simulink model "PubIfDecisionLM_MDL"  (R2020b)
settings: configuration reference "DspaceConfig" (kept outside this file)
PostLoadFcn:
  | if any(exist('dsrtsu_mdlpostloadfcn', 'file') ~= 0), dsrtsu_mdlpostloadfcn('Execute', bdroot); end
InitFcn:
  | , if any(exist('dsmpb_private', 'file') ~= 0), dsmpb_private('dsmpb_mdlclblib', 'Init', bdroot); end,
undefined symbols (not defined in the file or in its folder): OFM_OBJ_FUSIONTYPE_E, OFM_OBJ_MOVINGSTATE_E, OFM_OBJ_ORIENTATION_E, OFM_OBJ_TYPE_E, P_LM_Cyc, P_LM_EMLHistKapRcdBufSize, P_LM_EMLHistTrajBaseDis, P_LM_EMLHistTrajPNum, P_LM_EMLKapCorrMaxThre, P_LM_EMLMinKapThre, P_LM_EMLPathDisDiffThre, P_LM_EMLQuaFiltPar, P_LM_EMLTurnActKapThre, P_LM_EMLValidQuaThre, P_LM_FntPath1Disgap, P_LM_FntPath1MinDis, P_LM_FntPath1Timegap, P_LM_FntPath2Disgap, P_LM_FntPath2MinDis, P_LM_FntPath2Timegap, P_LM_FntPath3Disgap, P_LM_FntPath3MinDis, P_LM_FntPath3Timegap, P_LM_FusBLParFiltP, P_LM_FusEVDifC2Thre, P_LM_FusEVOPath1AllVSLDisThre, P_LM_FusEVOPath1AllVSLLostNumThre, P_LM_FusEVOPath1AllVSLQuaThre, P_LM_FusEVOPath1OTLFacNLC, P_LM_FusOTLQuaThre, P_LM_FusOTLSW, P_LM_FusParC0Index, P_LM_FusParC1Index, P_LM_FusParC2Index, P_LM_FusParC3Index, P_LM_FusVSLQuaThre, P_LM_FusVSLSW, P_LM_FusVSLValidSteerWheerAngThre, P_LM_FusVSLValidVxvThre, P_LM_LaneWidth, P_LM_OTLBufTPInfoEvaFactor, P_LM_OTLObjNum, P_LM_OTLObjSelectAgeThre, P_LM_OTLObjSelectDxAssessVx, P_LM_OTLObjSelectDxThre, P_LM_OTLObjSelectVxThre, P_LM_OTLObjSelectVyAssessDx, P_LM_OTLObjSelectVyThre, P_LM_OTLTrajPntBaseDis, P_LM_OTLTrajStdThre, P_LM_VSLAvailLineNum, P_LM_VSLBLSDiffThre, P_LM_VSLBLSDisRatio, P_LM_VSLFusBLParFiltP_C1, P_LM_VSLFusBLParFiltP_C2, P_LM_VSLFusBLParFiltP_C3, P_LM_VSLFusBLParFiltP_Quality, P_LM_VSLHistTrajBaseDis, P_LM_VSLHistTrajPNum, P_LM_VSLLCC0diff ... (+18)
libraries: simulink x145, LM_LIB x43
(part 16 of 24)

== system PubIfDecisionLM_MDL/Subsystem2/LM_OTL/LM_OTL_MovObjTrajRecord3/LM_OTL_ObjStoreInfoCalc/Subsystem/LM_OTL_BufLastTPInfo/Subsystem ==
  LM_OTLBufL1LastTPValidAdju : Inport
  LM_OTLBufL1LastPNumAdju : Inport  Port=2
  LM_OTLBufL1LastSPPosAdju : Inport  Port=3
  LM_OTLBufL1LastEPPosAdju : Inport  Port=4
  LM_OTLBufL2LastTPValidAdju : Inport  Port=5
  LM_OTLBufL2LastPNumAdju : Inport  Port=6
  LM_OTLBufL2LastSPPosAdju : Inport  Port=7
  LM_OTLBufL2LastEPPosAdju : Inport  Port=8
  LM_OTLBufE1LastTPValidAdju : Inport  Port=9
  LM_OTLBufE1LastPNumAdju : Inport  Port=10
  LM_OTLBufE1LastSPPosAdju : Inport  Port=11
  LM_OTLBufE1LastEPPosAdju : Inport  Port=12
  LM_OTLBufE2LastTPValidAdju : Inport  Port=13
  LM_OTLBufE2LastPNumAdju : Inport  Port=14
  LM_OTLBufE2LastSPPosAdju : Inport  Port=15
  LM_OTLBufE2LastEPPosAdju : Inport  Port=16
  LM_OTLBufR1LastTPValidAdju : Inport  Port=17
  LM_OTLBufR1LastPNumAdju : Inport  Port=18
  LM_OTLBufR1LastSPPosAdju : Inport  Port=19
  LM_OTLBufR1LastEPPosAdju : Inport  Port=20
  LM_OTLBufR2LastTPValidAdju : Inport  Port=21
  LM_OTLBufR2LastPNumAdju : Inport  Port=22
  LM_OTLBufR2LastSPPosAdju : Inport  Port=23
  LM_OTLBufR2LastEPPosAdju : Inport  Port=24
  Bus Creator{4,7..9} (4 alike) : BusCreator  Inputs=6
  LM_OTLBufLastTPValid : Outport
  LM_OTLBufLastPNumInfo : Outport  Port=2
  LM_OTLBufLastSPPosInfo : Outport  Port=3
  LM_OTLBufLastEPPosInfo : Outport  Port=4
  wires:
  Bus Creator4/1 -> LM_OTLBufLastTPValid/1  "LM_OTLBufLastTPValid"
  LM_OTLBufR2LastTPValidAdju/1 -> Bus Creator4/6  "LM_OTLBufR2LastTPValid"
  LM_OTLBufR1LastTPValidAdju/1 -> Bus Creator4/5  "LM_OTLBufR1LastTPValid"
  LM_OTLBufE2LastTPValidAdju/1 -> Bus Creator4/4  "LM_OTLBufE2LastTPValid"
  LM_OTLBufE1LastTPValidAdju/1 -> Bus Creator4/3  "LM_OTLBufE1LastTPValid"
  LM_OTLBufL2LastTPValidAdju/1 -> Bus Creator4/2  "LM_OTLBufL2LastTPValid"
  LM_OTLBufL1LastTPValidAdju/1 -> Bus Creator4/1  "LM_OTLBufL1LastTPValid"
  LM_OTLBufL1LastPNumAdju/1 -> Bus Creator7/1  "LM_OTLBufL1LastPNum"
  LM_OTLBufL2LastPNumAdju/1 -> Bus Creator7/2  "LM_OTLBufL2LastPNum"
  LM_OTLBufE1LastPNumAdju/1 -> Bus Creator7/3  "LM_OTLBufE1LastPNum"
  LM_OTLBufE2LastPNumAdju/1 -> Bus Creator7/4  "LM_OTLBufE2LastPNum"
  LM_OTLBufR1LastPNumAdju/1 -> Bus Creator7/5  "LM_OTLBufR1LastPNum"
  LM_OTLBufR2LastPNumAdju/1 -> Bus Creator7/6  "LM_OTLBufR2LastPNum"
  LM_OTLBufL1LastSPPosAdju/1 -> Bus Creator8/1  "LM_OTLBufL1LastSPPos"
  LM_OTLBufL2LastSPPosAdju/1 -> Bus Creator8/2  "LM_OTLBufL2LastSPPos"
  LM_OTLBufE1LastSPPosAdju/1 -> Bus Creator8/3  "LM_OTLBufE1LastSPPos"
  LM_OTLBufE2LastSPPosAdju/1 -> Bus Creator8/4  "LM_OTLBufE2LastSPPos"
  LM_OTLBufR1LastSPPosAdju/1 -> Bus Creator8/5  "LM_OTLBufR1LastSPPos"
  LM_OTLBufR2LastSPPosAdju/1 -> Bus Creator8/6  "LM_OTLBufR2LastSPPos"
  LM_OTLBufR2LastEPPosAdju/1 -> Bus Creator9/6  "LM_OTLBufR2LastEPPos"
  LM_OTLBufR1LastEPPosAdju/1 -> Bus Creator9/5  "LM_OTLBufR1LastEPPos"
  LM_OTLBufE2LastEPPosAdju/1 -> Bus Creator9/4  "LM_OTLBufE2LastEPPos"
  LM_OTLBufE1LastEPPosAdju/1 -> Bus Creator9/3  "LM_OTLBufE1LastEPPos"
  LM_OTLBufL2LastEPPosAdju/1 -> Bus Creator9/2  "LM_OTLBufL2LastEPPos"
  LM_OTLBufL1LastEPPosAdju/1 -> Bus Creator9/1  "LM_OTLBufL1LastEPPos"
  Bus Creator7/1 -> LM_OTLBufLastPNumInfo/1  "LM_OTLBufLastPNumInfo"
  Bus Creator8/1 -> LM_OTLBufLastSPPosInfo/1  "LM_OTLBufLastSPPosInfo"
  Bus Creator9/1 -> LM_OTLBufLastEPPosInfo/1  "LM_OTLBufLastEPPosInfo"

== system PubIfDecisionLM_MDL/Subsystem2/LM_VSL/LM_VSLFntPath/LM_VSL_LineInfoEvalutaion/LM_VSL_BaseLinePCalc3/Subsystem/Switch Case Action Subsystem ==
  LM_VSLLineMinQualityIndex : Inport
  LM_VSLLineC1Vect : Inport  Port=2
  LM_VSLLineC2Vect : Inport  Port=3
  LM_VSLLineC3Vect : Inport  Port=4
  LM_VSLLineQualityVect : Inport  Port=5
  LM_VSLMinQualityLineValid : Inport  Port=6
  LM_VSLLineDisFntVect : Inport  Port=7
  LM_VSLBLFntDis : Inport  Port=8
  Action Port : ActionPort  ActionPortLabel=case [ 2 ]:
  LM_VSLBaseParCalc : Subsystem
  LM_VSLLineQualitySumCalc : Subsystem
  LM_VSLBaseC1 : Outport
  LM_VSLBaseC2 : Outport  Port=2
  LM_VSLBaseC3 : Outport  Port=3
  LM_VSLBaseQuality : Outport  Port=4
  wires:
  LM_VSLLineQualitySumCalc/2(Diffnum) -> LM_VSLBaseParCalc/2(Diffnum)
  LM_VSLBLFntDis/1 -> LM_VSLLineQualitySumCalc/5(LM_VSLBLFntDis)
  LM_VSLLineDisFntVect/1 -> LM_VSLLineQualitySumCalc/4(LM_VSLLineDisFntVect)
  LM_VSLMinQualityLineValid/1 -> LM_VSLLineQualitySumCalc/3(LM_VSLMinQualityLineValid), LM_VSLBaseParCalc/5(LM_VSLMinQualityLineValid)
  LM_VSLBaseParCalc/3(LM_VSLBaseC3) -> LM_VSLBaseC3/1
  LM_VSLBaseParCalc/2(LM_VSLBaseC2) -> LM_VSLBaseC2/1
  LM_VSLBaseParCalc/1(LM_VSLBaseC1) -> LM_VSLBaseC1/1
  [LM_VSLLineMinQualityIndex] -> LM_VSLBaseParCalc/3(LM_VSLLineMinQualityIndex)
  LM_VSLLineC3Vect/1 -> LM_VSLBaseParCalc/8(LM_VSLLineC3Vect)
  LM_VSLLineC2Vect/1 -> LM_VSLBaseParCalc/7(LM_VSLLineC2Vect)
  LM_VSLLineC1Vect/1 -> LM_VSLBaseParCalc/6(LM_VSLLineC1Vect)
  LM_VSLLineQualitySumCalc/1(LM_VSLLineQualitySum) -> LM_VSLBaseParCalc/1(LM_VSLLineQualitySum)
  LM_VSLLineMinQualityIndex/1 -> LM_VSLLineQualitySumCalc/1(LM_VSLLineMinQualityIndex), [LM_VSLLineMinQualityIndex]
  LM_VSLLineQualityVect/1 -> LM_VSLLineQualitySumCalc/2(LM_VSLLineQualityVect), LM_VSLBaseParCalc/4(LM_VSLLineQualityVect)
  LM_VSLBaseParCalc/4(LM_VSLBaseQuality) -> LM_VSLBaseQuality/1

== system PubIfDecisionLM_MDL/Subsystem2/LM_VSL/LM_VSLFntPath/LM_VSL_LineInfoEvalutaion/LM_VSL_BaseLinePCalc3/Subsystem/Switch Case Action Subsystem1 ==
  Action Port : ActionPort  ActionPortLabel=case [ 4 ]:
  Constant{,1..3} (4 alike) : Constant  Value=0  OutDataTypeStr=single
  LM_VSLBaseC1 : Outport
  LM_VSLBaseC2 : Outport  Port=2
  LM_VSLBaseC3 : Outport  Port=3
  LM_VSLBaseQuality : Outport  Port=4
  wires:
  Constant2/1 -> LM_VSLBaseC3/1
  Constant1/1 -> LM_VSLBaseC2/1
  Constant/1 -> LM_VSLBaseC1/1
  Constant3/1 -> LM_VSLBaseQuality/1

== system PubIfDecisionLM_MDL/Subsystem2/LM_VSL/LM_VSLFntPath/LM_VSL_LineInfoEvalutaion/LM_VSL_BaseLinePCalc3/Subsystem/Switch Case Action Subsystem2 ==
  LM_VSLLineC1Vect : Inport
  LM_VSLLineC2Vect : Inport  Port=2
  LM_VSLLineC3Vect : Inport  Port=3
  LM_VSLLineQualityVect : Inport  Port=4
  LM_VSLLineMaxQualityIndex : Inport  Port=5
  Action Port : ActionPort  ActionPortLabel=case [ 3 ]:
  1-D Lookup Table : Lookup_n-D  NumberOfTableDimensions=1  BreakpointsForDimension1=P_LM_VSLAvailLineNum  Table=P_LM_VSLLineBaseQualityRatio  InternalRulePriority=Speed  RndMeth=Simplest  InputSameDT=on
  Constant1 : Constant  OutDataTypeStr=single
  Index Vector{,1..3} (4 alike) : MultiPortSwitch  Inputs=1
  Product : Product
  Saturation : Saturate  UpperLimit=4  LowerLimit=1
  LM_VSLBaseC1 : Outport
  LM_VSLBaseC2 : Outport  Port=2
  LM_VSLBaseC3 : Outport  Port=3
  LM_VSLBaseQuality : Outport  Port=4
  wires:
  Constant1/1 -> 1-D Lookup Table/1
  Product/1 -> LM_VSLBaseQuality/1
  1-D Lookup Table/1 -> Product/2
  Saturation/1 -> Index Vector/1, Index Vector1/1, Index Vector3/1, Index Vector2/1
  Index Vector2/1 -> LM_VSLBaseC3/1  "LM_VSLBaseC3"
  Index Vector/1 -> LM_VSLBaseC1/1  "LM_VSLBaseC1"
  Index Vector1/1 -> LM_VSLBaseC2/1  "LM_VSLBaseC2"
  LM_VSLLineMaxQualityIndex/1 -> Saturation/1
  LM_VSLLineC3Vect/1 -> Index Vector2/2
  LM_VSLLineC2Vect/1 -> Index Vector1/2
  LM_VSLLineC1Vect/1 -> Index Vector/2
  LM_VSLLineQualityVect/1 -> Index Vector3/2
  Index Vector3/1 -> Product/1  "LM_VSLBaseQuality"

== system PubIfDecisionLM_MDL/Subsystem2/LM_VSL/LM_VSLFntPath/LM_VSL_LineInfoEvalutaion/LM_VSL_BaseLinePCalc3/Subsystem/Switch Case Action Subsystem3 ==
  Diffnum : Inport
  LM_VSLDiffValid : Inport  Port=2
  LM_VSLLineMinQualityIndex : Inport  Port=3
  LM_VSLLineC1Vect : Inport  Port=4
  LM_VSLLineC2Vect : Inport  Port=5
  LM_VSLLineC3Vect : Inport  Port=6
  LM_VSLLineQualityVect : Inport  Port=7
  LM_VSLMinQualityLineValid : Inport  Port=8
  Action Port : ActionPort  ActionPortLabel=case [ 0 1 ]:
  LM_VSLBaseParCalc : Subsystem
  LM_VSLLineQualitySumCalc : Subsystem
  LM_VSLBaseC1 : Outport
  LM_VSLBaseC2 : Outport  Port=2
  LM_VSLBaseC3 : Outport  Port=3
  LM_VSLBaseQuality : Outport  Port=4
  wires:
  LM_VSLLineQualityVect/1 -> LM_VSLBaseParCalc/3(LM_VSLLineQualityVect), LM_VSLLineQualitySumCalc/2(LM_VSLLineQualityVect)
  LM_VSLLineMinQualityIndex/1 -> [LM_VSLLineMinQualityIndex], LM_VSLLineQualitySumCalc/1(LM_VSLLineMinQualityIndex)
  LM_VSLLineQualitySumCalc/1(LM_VSLLineQualitySum) -> LM_VSLBaseParCalc/1(LM_VSLLineQualitySum)
  LM_VSLLineC1Vect/1 -> LM_VSLBaseParCalc/7(LM_VSLLineC1Vect)
  LM_VSLLineC2Vect/1 -> LM_VSLBaseParCalc/8(LM_VSLLineC2Vect)
  LM_VSLLineC3Vect/1 -> LM_VSLBaseParCalc/9(LM_VSLLineC3Vect)
  [LM_VSLLineMinQualityIndex] -> LM_VSLBaseParCalc/2(LM_VSLLineMinQualityIndex)
  LM_VSLBaseParCalc/1(LM_VSLBaseC1) -> LM_VSLBaseC1/1
  LM_VSLBaseParCalc/2(LM_VSLBaseC2) -> LM_VSLBaseC2/1
  LM_VSLBaseParCalc/3(LM_VSLBaseC3) -> LM_VSLBaseC3/1
  LM_VSLMinQualityLineValid/1 -> LM_VSLBaseParCalc/4(LM_VSLMinQualityLineValid), LM_VSLLineQualitySumCalc/3(LM_VSLMinQualityLineValid)
  Diffnum/1 -> LM_VSLBaseParCalc/5(Diffnum), LM_VSLLineQualitySumCalc/4(Diffnum)
  LM_VSLDiffValid/1 -> LM_VSLBaseParCalc/6(LM_VSLDiffMaxValid), LM_VSLLineQualitySumCalc/5(LM_VSLDiffValidIndex)
  LM_VSLBaseParCalc/4(LM_VSLBaseQuality) -> LM_VSLBaseQuality/1

== system PubIfDecisionLM_MDL/Subsystem2/LM_VSL/LM_VSLFntPath/LM_VSL_LineInfoEvalutaion/LM_VSL_LineInfoEvalutaion/LM_VSL_LineDisEvaluation/If Action Subsystem ==
  Action Port : ActionPort  ActionPortLabel=if(u1 == 1)
  Constant : Constant  Value=0  OutDataTypeStr=single
  Constant1 : Constant  OutDataTypeStr=uint8
  Constant2 : Constant  Value=[1;2;3;4]  OutDataTypeStr=uint8
  Constant3 : Constant  Value=0  OutDataTypeStr=single
  LM_VSLLineMaxDis : Outport
  LM_VSLLineMaxDisIndex : Outport  Port=2
  LM_VSLLineDisSortIndexVect : Outport  Port=3
  LM_VSLLineMeanDis : Outport  Port=4
  wires:
  Constant3/1 -> LM_VSLLineMeanDis/1
  Constant/1 -> LM_VSLLineMaxDis/1
  Constant1/1 -> LM_VSLLineMaxDisIndex/1
  Constant2/1 -> LM_VSLLineDisSortIndexVect/1

== system PubIfDecisionLM_MDL/Subsystem2/LM_VSL/LM_VSLFntPath/LM_VSL_LineInfoEvalutaion/LM_VSL_LineInfoEvalutaion/LM_VSL_LineDisEvaluation/If Action Subsystem1 ==
  LM_VSLLineExistVect : Inport
  LM_VSLLineDisFntVect : Inport  Port=2
  Action Port : ActionPort  ActionPortLabel=else
  Constant2 : Constant  Value=[1;2;3;4]  OutDataTypeStr=uint8
  LM_VSLLineMaxDisCalc : MATLAB Function  TreatAsAtomicUnit=on
  Terminator : Terminator
  LM_VSLLineMaxDis : Outport
  LM_VSLLineMaxDisIndex : Outport  Port=2
  LM_VSLLineDisSortIndexVect : Outport  Port=3
  LM_VSLLineMeanDis : Outport  Port=4
  wires:
  LM_VSLLineMaxDisCalc/3(LM_VSLLineMeanDis) -> LM_VSLLineMeanDis/1
  LM_VSLLineDisFntVect/1 -> LM_VSLLineMaxDisCalc/1(LM_VSLLineDisFntVect)
  LM_VSLLineExistVect/1 -> Terminator/1
  LM_VSLLineMaxDisCalc/1(LM_VSLLineMaxDis) -> LM_VSLLineMaxDis/1
  LM_VSLLineMaxDisCalc/2(LM_VSLLineMaxDisIndex) -> LM_VSLLineMaxDisIndex/1
  Constant2/1 -> LM_VSLLineDisSortIndexVect/1

== system PubIfDecisionLM_MDL/Subsystem2/LM_VSL/LM_VSLFntPath/LM_VSL_LineInfoEvalutaion/LM_VSL_LineInfoEvalutaion/LM_VSL_LineQualityEvalutaion/If Action Subsystem ==
  Action Port : ActionPort  ActionPortLabel=if(u1 == 1)
  Constant{,3,5..6} (4 alike) : Constant  Value=0  OutDataTypeStr=single
  Constant1 : Constant  OutDataTypeStr=uint8
  Constant4 : Constant  OutDataTypeStr=uint8
  LM_VSLLineMaxQuality : Outport
  LM_VSLLineMaxQualityIndex : Outport  Port=2
  LM_VSLLineMinQualityIndex : Outport  Port=3
  LM_VSLLineMinQuality : Outport  Port=4
  LM_VSLLineMeanQuality : Outport  Port=5
  LM_VSLLineQualityVar : Outport  Port=6
  wires:
  Constant/1 -> LM_VSLLineMaxQuality/1
  Constant1/1 -> LM_VSLLineMaxQualityIndex/1
  Constant3/1 -> LM_VSLLineMinQuality/1
  Constant4/1 -> LM_VSLLineMinQualityIndex/1
  Constant5/1 -> LM_VSLLineMeanQuality/1
  Constant6/1 -> LM_VSLLineQualityVar/1

== system PubIfDecisionLM_MDL/Subsystem2/LM_VSL/LM_VSLFntPath/LM_VSL_LineInfoEvalutaion/LM_VSL_LineInfoEvalutaion/LM_VSL_LineQualityEvalutaion/If Action Subsystem1 ==
  LM_VSLLineExistVect : Inport
  LM_VSLLineQualityVect : Inport  Port=2
  Action Port : ActionPort  ActionPortLabel=else
  Data Type Conversion : DataTypeConversion
  For Iterator Subsystem : Subsystem  TreatAsAtomicUnit=on
  LM_VSL_LineQualityEvaluation : MATLAB Function  TreatAsAtomicUnit=on
  Terminator : Terminator
  Terminator1 : Terminator
  LM_VSLLineMaxQuality : Outport
  LM_VSLLineMaxQualityIndex : Outport  Port=2
  LM_VSLLineMinQualityIndex : Outport  Port=3
  LM_VSLLineMinQuality : Outport  Port=4
  LM_VSLLineMeanQuality : Outport  Port=5
  LM_VSLLineQualityVar : Outport  Port=6
  wires:
  LM_VSL_LineQualityEvaluation/4(LM_VSLLineMinQualiyIndex) -> Terminator1/1
  LM_VSL_LineQualityEvaluation/3(LM_VSLLineMinQualiy) -> Terminator/1
  Data Type Conversion/1 -> LM_VSLLineMinQualityIndex/1
  LM_VSLLineExistVect/1 -> LM_VSL_LineQualityEvaluation/1(LM_VSLLineExistVect)
  LM_VSL_LineQualityEvaluation/1(LM_VSLLineMaxQualiy) -> LM_VSLLineMaxQuality/1
  LM_VSL_LineQualityEvaluation/2(LM_VSLLineMaxQualiyIndex) -> LM_VSLLineMaxQualityIndex/1
  LM_VSL_LineQualityEvaluation/5(LM_VSLLineMeanQuality) -> LM_VSLLineMeanQuality/1
  LM_VSL_LineQualityEvaluation/6(LM_VSLLineQualityVar) -> LM_VSLLineQualityVar/1
  LM_VSLLineQualityVect/1 -> For Iterator Subsystem/1(LM_VSLLineQualityVect), LM_VSL_LineQualityEvaluation/2(LM_VSLLineQualityVect)
  For Iterator Subsystem/2(LM_VSLLineMinQualityIndex) -> Data Type Conversion/1
  For Iterator Subsystem/1(LM_VSLLineMinQuality) -> LM_VSLLineMinQuality/1

== system PubIfDecisionLM_MDL/Subsystem2/LM_VSL/LM_VSLFntPath/LM_VSL_LineInfoEvalutaion/LM_VSL_LineInfoEvalutaion/LM_VSL_LineQualityEvalutaion/LM_VSLMinQualityLineValidJudge ==
  LM_VSLLineMinQuality : Inport
  LM_VSLLineMeanQuality : Inport  Port=2
  Constant : Constant  Value=P_LM_VSLLineQualitydiffThre  OutDataTypeStr=single
  Constant1 : Constant  Value=P_LM_VSLLineMinQualityThre  OutDataTypeStr=single
  Logical Operator : Logic  AllPortsSameDT=off  OutDataTypeStr=boolean
  Relational Operator : RelationalOperator  Operator=<=  OutDataTypeStr=boolean  RndMeth=Nearest
  Relational Operator1 : RelationalOperator  Operator=>  OutDataTypeStr=boolean  RndMeth=Nearest
  Subtract : Sum  Inputs=+-
  LM_VSLMinQualityLineValid : Outport
  wires:
  LM_VSLLineMeanQuality/1 -> Subtract/1
  LM_VSLLineMinQuality/1 -> Relational Operator1/1, Subtract/2
  Subtract/1 -> Relational Operator/1
  Constant/1 -> Relational Operator/2
  Relational Operator/1 -> Logical Operator/1
  Constant1/1 -> Relational Operator1/2
  Relational Operator1/1 -> Logical Operator/2
  Logical Operator/1 -> LM_VSLMinQualityLineValid/1  "LM_VSLMinQualityLineValid"

== system PubIfDecisionLM_MDL/Subsystem2/LM_VSL/LM_VSLRearPath/LM_VSLHistLineInfoCoordinateConvert/If Action Subsystem/For Each Subsystem/LM_VSL_LRC0HistInfoConvert ==
  LM_VSLLRC0HistInfoXK1 : Inport
  LM_VSLLRC0HistInfoYK1 : Inport  Port=2
  LM_EgoVehOffsetX : Inport  Port=3
  LM_EgoVehOffsetY : Inport  Port=4
  LM_EgoVehOffsetAng : Inport  Port=5
  Add : Sum
  Product{,1..3} (4 alike) : Product
  Sin : Trigonometry
  Sin1 : Trigonometry  Operator=cos
  Subtract : Sum  Inputs=+-
  Subtract1 : Sum  Inputs=+-
  Subtract2 : Sum  Inputs=+-
  LM_VSLLLC0HistInfoXK1Adju : Outport
  LM_VSLLLC0HistInfoYK1Adju : Outport  Port=2
  wires:
  Subtract2/1 -> LM_VSLLLC0HistInfoXK1Adju/1  "LM_VSLLLC0HistInfoXK1Adju"
  LM_EgoVehOffsetX/1 -> Subtract/2
  LM_EgoVehOffsetY/1 -> Subtract1/2
  LM_VSLLRC0HistInfoXK1/1 -> Subtract/1
  Add/1 -> LM_VSLLLC0HistInfoYK1Adju/1  "LM_VSLLLC0HistInfoYK1Adju"
  Product3/1 -> Add/2
  Subtract/1 -> Product/1, Product2/1
  Sin/1 -> Product1/2, Product2/2
  LM_EgoVehOffsetAng/1 -> Sin/1, Sin1/1
  LM_VSLLRC0HistInfoYK1/1 -> Subtract1/1
  Product1/1 -> Subtract2/2
  Product/1 -> Subtract2/1
  Product2/1 -> Add/1
  Sin1/1 -> Product/2, Product3/2
  Subtract1/1 -> Product1/1, Product3/1

== system PubIfDecisionLM_MDL/Subsystem2/LM_VSL/LM_VSLRearPath/LM_VSLHistLineInfoCoordinateConvert/If Action Subsystem/For Each Subsystem/LM_VSL_RLC0HistInfoConvert ==
  LM_VSLRLC0HistInfoXK1 : Inport
  LM_VSLRLC0HistInfoYK1 : Inport  Port=2
  LM_EgoVehOffsetX : Inport  Port=3
  LM_EgoVehOffsetY : Inport  Port=4
  LM_EgoVehOffsetAng : Inport  Port=5
  Add : Sum
  Product{,1..3} (4 alike) : Product
  Sin : Trigonometry
  Sin1 : Trigonometry  Operator=cos
  Subtract : Sum  Inputs=+-
  Subtract1 : Sum  Inputs=+-
  Subtract2 : Sum  Inputs=+-
  LM_VSLLLC0HistInfoXK1Adju : Outport
  LM_VSLLLC0HistInfoYK1Adju : Outport  Port=2
  wires:
  Subtract1/1 -> Product3/1, Product1/1
  Sin1/1 -> Product3/2, Product/2
  Product2/1 -> Add/1
  Product/1 -> Subtract2/1
  Product1/1 -> Subtract2/2
  LM_VSLRLC0HistInfoYK1/1 -> Subtract1/1
  LM_EgoVehOffsetAng/1 -> Sin1/1, Sin/1
  Sin/1 -> Product2/2, Product1/2
  Subtract/1 -> Product2/1, Product/1
  Product3/1 -> Add/2
  Add/1 -> LM_VSLLLC0HistInfoYK1Adju/1  "LM_VSLLLC0HistInfoYK1Adju"
  LM_VSLRLC0HistInfoXK1/1 -> Subtract/1
  LM_EgoVehOffsetY/1 -> Subtract1/2
  LM_EgoVehOffsetX/1 -> Subtract/2
  Subtract2/1 -> LM_VSLLLC0HistInfoXK1Adju/1  "LM_VSLLLC0HistInfoXK1Adju"

== system PubIfDecisionLM_MDL/Subsystem2/DIR/DrivingIntentionRecognition1/DIR_LaneChangeProbCalc/DIR_LaneChangeLeftProbCalc/If Action Subsystem/DIR_LaneChgLeProbByLaneInfo/DIR_LaneC0DifCalc ==
  DIR_LaneC0DifK1 : Inport
  LM_LRC0 : Inport  Port=2
  LM_RLC0 : Inport  Port=3
  Abs : Abs
  Add : Sum
  Add1 : Sum
  Constant : Constant  Value=0.5  OutDataTypeStr=single
  Product : Product
  Subtract : Sum  Inputs=+-
  DIR_LaneC0Dif : Outport
  wires:
  Abs/1 -> Subtract/1
  Product/1 -> Add1/1
  Add/1 -> Abs/1
  LM_LRC0/1 -> Add/1
  LM_RLC0/1 -> Add/2
  DIR_LaneC0DifK1/1 -> Add1/2, Subtract/2
  Subtract/1 -> Product/1
  Constant/1 -> Product/2
  Add1/1 -> DIR_LaneC0Dif/1

== system PubIfDecisionLM_MDL/Subsystem2/DIR/DrivingIntentionRecognition1/DIR_LaneChangeProbCalc/DIR_LaneChangeLeftProbCalc/If Action Subsystem/DIR_LaneChgLeProbByLaneInfo/DIR_LaneChgLeProbCalcByLaneBorder ==
  DIR_LaneC0Dif : Inport
  LM_LRC0 : Inport  Port=2
  1-D Lookup Table : Lookup_n-D  NumberOfTableDimensions=1  BreakpointsForDimension1=single([0.7,0.79,0.88,0.97,1.06,1.15]);  Table=single([0,0.2,0.4,0.6,0.8,1]);  InternalRulePriority=Speed  RndMeth=Simplest  InputSameDT=on
  Constant : Constant  Value=1.15  OutDataTypeStr=single
  Constant1 : Constant  OutDataTypeStr=single
  Constant2 : Constant  Value=0.7  OutDataTypeStr=single
  Constant3 : Constant  Value=0  OutDataTypeStr=single
  Constant4 : Constant  Value=1.7  OutDataTypeStr=single
  Logical Operator : Logic  Inputs=3  AllPortsSameDT=off  OutDataTypeStr=boolean
  Logical Operator1 : Logic  AllPortsSameDT=off  OutDataTypeStr=boolean
  Relational Operator : RelationalOperator  OutDataTypeStr=boolean  RndMeth=Simplest
  Relational Operator1 : RelationalOperator  Operator=<  OutDataTypeStr=boolean  RndMeth=Simplest
  Relational Operator2 : RelationalOperator  OutDataTypeStr=boolean  RndMeth=Simplest
  Relational Operator3 : RelationalOperator  Operator=<  OutDataTypeStr=boolean  RndMeth=Simplest
  Switch : Switch  Criteria=u2 ~= 0
  Switch1 : Switch  Criteria=u2 ~= 0
  DIR_LC2LeProbByLaneBorder : Outport
  wires:
  Constant/1 -> Relational Operator/2, Relational Operator1/2
  Relational Operator/1 -> Logical Operator1/2
  Constant1/1 -> Switch/1
  Relational Operator1/1 -> Logical Operator/2
  Constant2/1 -> Relational Operator2/2
  Relational Operator2/1 -> Logical Operator/3
  Logical Operator/1 -> Switch1/2
  Switch1/1 -> Switch/3
  Constant3/1 -> Switch1/3
  Switch/1 -> DIR_LC2LeProbByLaneBorder/1  "DIR_LC2LeProbByLaneBorder"
  DIR_LaneC0Dif/1 -> 1-D Lookup Table/1, Relational Operator2/1, Relational Operator1/1, Relational Operator/1
  1-D Lookup Table/1 -> Switch1/1
  LM_LRC0/1 -> Relational Operator3/1
  Constant4/1 -> Relational Operator3/2
  Relational Operator3/1 -> Logical Operator/1, Logical Operator1/1
  Logical Operator1/1 -> Switch/2

== system PubIfDecisionLM_MDL/Subsystem2/DIR/DrivingIntentionRecognition1/DIR_LaneChangeProbCalc/DIR_LaneChangeLeftProbCalc/If Action Subsystem/DIR_LaneChgLeProbCalcBySteer/DIR_LaneChg2LeftProbCalcBySteer ==
  DIR_LC2LeProbBySteerWheelAng : Inport
  DIR_LC2LeProbBytTurnLamp : Inport  Port=2
  Max : MinMax  Function=max  Inputs=2
  DIR_LC2LeProbBySteer : Outport
  wires:
  DIR_LC2LeProbBySteerWheelAng/1 -> Max/1
  DIR_LC2LeProbBytTurnLamp/1 -> Max/2
  Max/1 -> DIR_LC2LeProbBySteer/1  "DIR_LC2LeProbBySteer"

== system PubIfDecisionLM_MDL/Subsystem2/DIR/DrivingIntentionRecognition1/DIR_LaneChangeProbCalc/DIR_LaneChangeLeftProbCalc/If Action Subsystem/DIR_LaneChgLeProbCalcBySteer/DIR_LaneChg2LeftProbCalcBySteerWheelAng ==
  SteerWheelAngle : Inport
  SteerWheelAngleSign : Inport  Port=2
  1-D Lookup Table : Lookup_n-D  NumberOfTableDimensions=1  BreakpointsForDimension1=single([9,15,20,25]);  Table=single([0,0.33000001311302185,0.6700000166893005,1]);  InternalRulePriority=Speed  RndMeth=Simplest  InputSameDT=on
  Constant : Constant  Value=25  OutDataTypeStr=single
  Constant1 : Constant  OutDataTypeStr=single
  Constant2 : Constant  Value=9  OutDataTypeStr=single
  Constant3 : Constant  Value=0  OutDataTypeStr=single
  Constant4 : Constant  Value=0  OutDataTypeStr=uint8
  Display{,1..3} (4 alike) : Display
  Logical Operator : Logic  Inputs=3  AllPortsSameDT=off  OutDataTypeStr=boolean
  Logical Operator1 : Logic  AllPortsSameDT=off  OutDataTypeStr=boolean
  Relational Operator : RelationalOperator  OutDataTypeStr=boolean  RndMeth=Simplest
  Relational Operator1 : RelationalOperator  Operator=<  OutDataTypeStr=boolean  RndMeth=Simplest
  Relational Operator2 : RelationalOperator  OutDataTypeStr=boolean  RndMeth=Simplest
  Relational Operator3 : RelationalOperator  Operator===  OutDataTypeStr=boolean  RndMeth=Simplest
  Switch : Switch  Criteria=u2 ~= 0
  Switch1 : Switch  Criteria=u2 ~= 0
  DIR_LC2LeProbBySteerWheelAng : Outport
  wires:
  1-D Lookup Table/1 -> Display/1, Switch1/1
  Constant/1 -> Relational Operator/2, Relational Operator1/2
  SteerWheelAngle/1 -> 1-D Lookup Table/1, Relational Operator2/1, Relational Operator1/1, Relational Operator/1
  Switch1/1 -> Display1/1, Switch/3
  Constant2/1 -> Relational Operator2/2
  Logical Operator/1 -> Display2/1, Switch1/2
  Constant3/1 -> Switch1/3
  Relational Operator1/1 -> Logical Operator/1
  Relational Operator2/1 -> Logical Operator/2
  Switch/1 -> DIR_LC2LeProbBySteerWheelAng/1  "DIR_LC2LeProbBySteerWheelAng"
  Constant1/1 -> Switch/1
  Logical Operator1/1 -> Switch/2
  SteerWheelAngleSign/1 -> Relational Operator3/1
  Relational Operator3/1 -> Display3/1, [SteerLeftFlg], Logical Operator1/1
  [SteerLeftFlg] -> Logical Operator/3
  Relational Operator/1 -> Logical Operator1/2
  Constant4/1 -> Relational Operator3/2

== system PubIfDecisionLM_MDL/Subsystem2/DIR/DrivingIntentionRecognition1/DIR_LaneChangeProbCalc/DIR_LaneChangeLeftProbCalc/If Action Subsystem/DIR_LaneChgLeProbCalcBySteer/DIR_LaneChg2LeftProbCalcByTurnLampOnTime ==
  DIR_LeftTurnLampOnTime : Inport
  1-D Lookup Table : Lookup_n-D  NumberOfTableDimensions=1  BreakpointsForDimension1=single([0,0.30000001192092896,0.6000000238418579,0.8999999761581421,1.2000000476837158,1.5]);  Table=single([0,0.20000000298023224,0.4000000059604645,0.6000000238418579,0.800000011920929,1]);  InternalRulePriority=Speed  RndMeth=Simplest  InputSameDT=on
  Constant : Constant  Value=1.5  OutDataTypeStr=single
  Constant1 : Constant  OutDataTypeStr=single
  Constant2 : Constant  Value=0  OutDataTypeStr=single
  Constant3 : Constant  Value=0  OutDataTypeStr=single
  Logical Operator : Logic  AllPortsSameDT=off  OutDataTypeStr=boolean
  Relational Operator : RelationalOperator  OutDataTypeStr=boolean  RndMeth=Simplest
  Relational Operator1 : RelationalOperator  Operator=<  OutDataTypeStr=boolean  RndMeth=Simplest
  Relational Operator2 : RelationalOperator  Operator=>  OutDataTypeStr=boolean  RndMeth=Simplest
  Switch : Switch  Criteria=u2 ~= 0
  Switch1 : Switch  Criteria=u2 ~= 0
  DIR_LC2LeProbBytTurnLamp : Outport
  wires:
  DIR_LeftTurnLampOnTime/1 -> 1-D Lookup Table/1, Relational Operator2/1, Relational Operator1/1, Relational Operator/1
  Constant/1 -> Relational Operator1/2, Relational Operator/2
  Relational Operator/1 -> Switch/2
  Constant1/1 -> Switch/1
  Constant2/1 -> Relational Operator2/2
  Relational Operator1/1 -> Logical Operator/1
  Relational Operator2/1 -> Logical Operator/2
  Logical Operator/1 -> Switch1/2
  Constant3/1 -> Switch1/3
  Switch1/1 -> Switch/3
  Switch/1 -> DIR_LC2LeProbBytTurnLamp/1  "DIR_LC2LeProbBytTurnLamp"
  1-D Lookup Table/1 -> Switch1/1

== system PubIfDecisionLM_MDL/Subsystem2/DIR/DrivingIntentionRecognition1/DIR_LaneChangeProbCalc/DIR_LaneChangeLeftProbCalc/If Action Subsystem1/DIR_LaneChgLeProbCalcBySteer/If Action Subsystem ==
  SteerWheelAngle : Inport
  SteerWheelAngleSign : Inport  Port=2
  vxvRefMs : Inport  Port=3
  Action Port : ActionPort  ActionPortLabel=if(u1 ~= 0)
  Constant1 : Constant  Value=0  OutDataTypeStr=single
  Constant2 : Constant  Value=3.5  OutDataTypeStr=single
  Constant4 : Constant  Value=0  OutDataTypeStr=uint8
  Logical Operator1 : Logic  Inputs=3  AllPortsSameDT=off  OutDataTypeStr=boolean
  Relational Operator : RelationalOperator  OutDataTypeStr=boolean  RndMeth=Simplest
  Relational Operator1 : RelationalOperator  Operator=>  OutDataTypeStr=boolean  RndMeth=Simplest
  Relational Operator3 : RelationalOperator  Operator===  OutDataTypeStr=boolean  RndMeth=Simplest
  DIR_LaneChgLeBySteerValid : Outport
  wires:
  Constant4/1 -> Relational Operator3/2
  Relational Operator3/1 -> Logical Operator1/1
  SteerWheelAngle/1 -> Relational Operator/1
  SteerWheelAngleSign/1 -> Relational Operator3/1
  Relational Operator/1 -> Logical Operator1/2
  vxvRefMs/1 -> Relational Operator1/1
  Constant2/1 -> Relational Operator/2
  Logical Operator1/1 -> DIR_LaneChgLeBySteerValid/1  "DIR_LaneChgLeBySteerValid"
  Constant1/1 -> Relational Operator1/2
  Relational Operator1/1 -> Logical Operator1/3

== system PubIfDecisionLM_MDL/Subsystem2/DIR/DrivingIntentionRecognition1/DIR_LaneChangeProbCalc/DIR_LaneChangeLeftProbCalc/If Action Subsystem1/DIR_LaneChgLeProbCalcBySteer/If Action Subsystem1 ==
  SteerWheelAngle : Inport
  SteerWheelAngleSign : Inport  Port=2
  vxvRefMs : Inport  Port=3
  Action Port : ActionPort  ActionPortLabel=else
  1-D Lookup Table : Lookup_n-D  NumberOfTableDimensions=1  BreakpointsForDimension1=single([5,15,25,35]);  Table=single([10,9,6,3]);  InternalRulePriority=Speed  RndMeth=Simplest  InputSameDT=on
  Constant1 : Constant  Value=0  OutDataTypeStr=single
  Constant4 : Constant  Value=0  OutDataTypeStr=uint8
  Logical Operator1 : Logic  Inputs=3  AllPortsSameDT=off  OutDataTypeStr=boolean
  Relational Operator : RelationalOperator  OutDataTypeStr=boolean  RndMeth=Simplest
  Relational Operator2 : RelationalOperator  Operator=>  OutDataTypeStr=boolean  RndMeth=Simplest
  Relational Operator3 : RelationalOperator  Operator===  OutDataTypeStr=boolean  RndMeth=Simplest
  DIR_LaneChgLeBySteerValid : Outport
  wires:
  Logical Operator1/1 -> DIR_LaneChgLeBySteerValid/1  "DIR_LaneChgLeBySteerValid"
  Constant4/1 -> Relational Operator3/2
  1-D Lookup Table/1 -> Relational Operator/2
  SteerWheelAngleSign/1 -> Relational Operator3/1
  SteerWheelAngle/1 -> Relational Operator/1
  Relational Operator/1 -> Logical Operator1/2
  Relational Operator3/1 -> Logical Operator1/1
  vxvRefMs/1 -> Relational Operator2/1, 1-D Lookup Table/1
  Constant1/1 -> Relational Operator2/2
  Relational Operator2/1 -> Logical Operator1/3

== system PubIfDecisionLM_MDL/Subsystem2/DIR/DrivingIntentionRecognition1/DIR_LaneChangeProbCalc/DIR_LaneChangeRightProbCalc/If Action Subsystem/DIR_LaneChgLeProbByLaneInfo/DIR_LaneC0DifCalc ==
  DIR_LaneC0DifK1 : Inport
  LM_LRC0 : Inport  Port=2
  LM_RLC0 : Inport  Port=3
  Abs : Abs
  Add : Sum
  Add1 : Sum
  Constant : Constant  Value=0.5  OutDataTypeStr=single
  Product : Product
  Subtract : Sum  Inputs=+-
  DIR_LaneC0Dif : Outport
  wires:
  Add1/1 -> DIR_LaneC0Dif/1
  Constant/1 -> Product/2
  Subtract/1 -> Product/1
  DIR_LaneC0DifK1/1 -> Subtract/2, Add1/2
  LM_RLC0/1 -> Add/2
  LM_LRC0/1 -> Add/1
  Add/1 -> Abs/1
  Product/1 -> Add1/1
  Abs/1 -> Subtract/1

== system PubIfDecisionLM_MDL/Subsystem2/DIR/DrivingIntentionRecognition1/DIR_LaneChangeProbCalc/DIR_LaneChangeRightProbCalc/If Action Subsystem/DIR_LaneChgLeProbByLaneInfo/DIR_LaneChgLeProbCalcByLaneBorder ==
  DIR_LaneC0Dif : Inport
  LM_LRC0 : Inport  Port=2
  1-D Lookup Table : Lookup_n-D  NumberOfTableDimensions=1  BreakpointsForDimension1=single([0.7,0.79,0.88,0.97,1.06,1.15]);  Table=single([0,0.2,0.4,0.6,0.8,1]);  InternalRulePriority=Speed  RndMeth=Simplest  InputSameDT=on
  Constant : Constant  Value=1.15  OutDataTypeStr=single
  Constant1 : Constant  OutDataTypeStr=single
  Constant2 : Constant  Value=0.7  OutDataTypeStr=single
  Constant3 : Constant  Value=0  OutDataTypeStr=single
  Constant4 : Constant  Value=1.7  OutDataTypeStr=single
  Logical Operator : Logic  Inputs=3  AllPortsSameDT=off  OutDataTypeStr=boolean
  Logical Operator1 : Logic  AllPortsSameDT=off  OutDataTypeStr=boolean
  Relational Operator : RelationalOperator  OutDataTypeStr=boolean  RndMeth=Simplest
  Relational Operator1 : RelationalOperator  Operator=<  OutDataTypeStr=boolean  RndMeth=Simplest
  Relational Operator2 : RelationalOperator  OutDataTypeStr=boolean  RndMeth=Simplest
  Relational Operator3 : RelationalOperator  Operator=<  OutDataTypeStr=boolean  RndMeth=Simplest
  Switch : Switch  Criteria=u2 ~= 0
  Switch1 : Switch  Criteria=u2 ~= 0
  DIR_LC2RigProbByLaneBorder : Outport
  wires:
  Logical Operator1/1 -> Switch/2
  Relational Operator3/1 -> Logical Operator1/1, Logical Operator/1
  Constant4/1 -> Relational Operator3/2
  LM_LRC0/1 -> Relational Operator3/1
  1-D Lookup Table/1 -> Switch1/1
  DIR_LaneC0Dif/1 -> Relational Operator/1, Relational Operator1/1, Relational Operator2/1, 1-D Lookup Table/1
  Switch/1 -> DIR_LC2RigProbByLaneBorder/1  "DIR_LC2RigProbByLaneBorder"
  Constant3/1 -> Switch1/3
  Switch1/1 -> Switch/3
  Logical Operator/1 -> Switch1/2
  Relational Operator2/1 -> Logical Operator/3
  Constant2/1 -> Relational Operator2/2
  Relational Operator1/1 -> Logical Operator/2
  Constant1/1 -> Switch/1
  Relational Operator/1 -> Logical Operator1/2
  Constant/1 -> Relational Operator1/2, Relational Operator/2

== system PubIfDecisionLM_MDL/Subsystem2/DIR/DrivingIntentionRecognition1/DIR_LaneChangeProbCalc/DIR_LaneChangeRightProbCalc/If Action Subsystem/DIR_LaneChgLeProbCalcBySteer/DIR_LaneChg2LeftProbCalcBySteer ==
  DIR_LC2RigProbBySteerWheelAng : Inport
  DIR_LC2RigProbBytTurnLamp : Inport  Port=2
  Max : MinMax  Function=max  Inputs=2
  DIR_LC2RigProbBySteer : Outport
  wires:
  Max/1 -> DIR_LC2RigProbBySteer/1  "DIR_LC2RigProbBySteer"
  DIR_LC2RigProbBytTurnLamp/1 -> Max/2
  DIR_LC2RigProbBySteerWheelAng/1 -> Max/1

== system PubIfDecisionLM_MDL/Subsystem2/DIR/DrivingIntentionRecognition1/DIR_LaneChangeProbCalc/DIR_LaneChangeRightProbCalc/If Action Subsystem/DIR_LaneChgLeProbCalcBySteer/DIR_LaneChg2LeftProbCalcBySteerWheelAng ==
  SteerWheelAngle : Inport
  SteerWheelAngleSign : Inport  Port=2
  1-D Lookup Table : Lookup_n-D  NumberOfTableDimensions=1  BreakpointsForDimension1=single([9,15,20,25]);  Table=single([0,0.33000001311302185,0.6700000166893005,1]);  InternalRulePriority=Speed  RndMeth=Simplest  InputSameDT=on
  Constant : Constant  Value=25  OutDataTypeStr=single
  Constant1 : Constant  OutDataTypeStr=single
  Constant2 : Constant  Value=9  OutDataTypeStr=single
  Constant3 : Constant  Value=0  OutDataTypeStr=single
  Constant4 : Constant  Value=0  OutDataTypeStr=uint8
  Display{,1..3} (4 alike) : Display
  Logical Operator : Logic  Inputs=3  AllPortsSameDT=off  OutDataTypeStr=boolean
  Logical Operator1 : Logic  AllPortsSameDT=off  OutDataTypeStr=boolean
  Relational Operator : RelationalOperator  OutDataTypeStr=boolean  RndMeth=Simplest
  Relational Operator1 : RelationalOperator  Operator=<  OutDataTypeStr=boolean  RndMeth=Simplest
  Relational Operator2 : RelationalOperator  OutDataTypeStr=boolean  RndMeth=Simplest
  Relational Operator3 : RelationalOperator  Operator===  OutDataTypeStr=boolean  RndMeth=Simplest
  Switch : Switch  Criteria=u2 ~= 0
  Switch1 : Switch  Criteria=u2 ~= 0
  DIR_LC2RigProbBySteerWheelAng : Outport
  wires:
  Constant4/1 -> Relational Operator3/2
  Relational Operator/1 -> Logical Operator1/2
  [SteerLeftFlg] -> Logical Operator/3
  Relational Operator3/1 -> Logical Operator1/1, [SteerLeftFlg], Display3/1
  SteerWheelAngleSign/1 -> Relational Operator3/1
  Logical Operator1/1 -> Switch/2
  Constant1/1 -> Switch/1
  Switch/1 -> DIR_LC2RigProbBySteerWheelAng/1  "DIR_LC2RigProbBySteerWheelAng"
  Relational Operator2/1 -> Logical Operator/2
  Relational Operator1/1 -> Logical Operator/1
  Constant3/1 -> Switch1/3
  Logical Operator/1 -> Switch1/2, Display2/1
  Constant2/1 -> Relational Operator2/2
  Switch1/1 -> Switch/3, Display1/1
  SteerWheelAngle/1 -> Relational Operator/1, Relational Operator1/1, Relational Operator2/1, 1-D Lookup Table/1
  Constant/1 -> Relational Operator1/2, Relational Operator/2
  1-D Lookup Table/1 -> Switch1/1, Display/1

== system PubIfDecisionLM_MDL/Subsystem2/DIR/DrivingIntentionRecognition1/DIR_LaneChangeProbCalc/DIR_LaneChangeRightProbCalc/If Action Subsystem/DIR_LaneChgLeProbCalcBySteer/DIR_LaneChg2LeftProbCalcByTurnLampOnTime ==
  DIR_RightTurnLampOnTime : Inport
  1-D Lookup Table : Lookup_n-D  NumberOfTableDimensions=1  BreakpointsForDimension1=single([0,0.30000001192092896,0.6000000238418579,0.8999999761581421,1.2000000476837158,1.5]);  Table=single([0,0.20000000298023224,0.4000000059604645,0.6000000238418579,0.800000011920929,1]);  InternalRulePriority=Speed  RndMeth=Simplest  InputSameDT=on
  Constant : Constant  Value=1.5  OutDataTypeStr=single
  Constant1 : Constant  OutDataTypeStr=single
  Constant2 : Constant  Value=0  OutDataTypeStr=single
  Constant3 : Constant  Value=0  OutDataTypeStr=single
  Logical Operator : Logic  AllPortsSameDT=off  OutDataTypeStr=boolean
  Relational Operator : RelationalOperator  OutDataTypeStr=boolean  RndMeth=Simplest
  Relational Operator1 : RelationalOperator  Operator=<  OutDataTypeStr=boolean  RndMeth=Simplest
  Relational Operator2 : RelationalOperator  Operator=>  OutDataTypeStr=boolean  RndMeth=Simplest
  Switch : Switch  Criteria=u2 ~= 0
  Switch1 : Switch  Criteria=u2 ~= 0
  DIR_LC2RigProbBytTurnLamp : Outport
  wires:
  1-D Lookup Table/1 -> Switch1/1
  Switch/1 -> DIR_LC2RigProbBytTurnLamp/1  "DIR_LC2RigProbBytTurnLamp"
  Switch1/1 -> Switch/3
  Constant3/1 -> Switch1/3
  Logical Operator/1 -> Switch1/2
  Relational Operator2/1 -> Logical Operator/2
  Relational Operator1/1 -> Logical Operator/1
  Constant2/1 -> Relational Operator2/2
  Constant1/1 -> Switch/1
  Relational Operator/1 -> Switch/2
  Constant/1 -> Relational Operator/2, Relational Operator1/2
  DIR_RightTurnLampOnTime/1 -> Relational Operator/1, Relational Operator1/1, Relational Operator2/1, 1-D Lookup Table/1

== system PubIfDecisionLM_MDL/Subsystem2/DIR/DrivingIntentionRecognition1/DIR_LaneChangeProbCalc/DIR_LaneChangeRightProbCalc/If Action Subsystem1/DIR_LaneChgLeProbCalcBySteer/If Action Subsystem ==
  SteerWheelAngle : Inport
  SteerWheelAngleSign : Inport  Port=2
  vxvRefMs : Inport  Port=3
  Action Port : ActionPort  ActionPortLabel=if(u1 ~= 0)
  Constant1 : Constant  Value=0  OutDataTypeStr=single
  Constant2 : Constant  Value=3.5  OutDataTypeStr=single
  Constant4 : Constant  OutDataTypeStr=uint8
  Logical Operator1 : Logic  Inputs=3  AllPortsSameDT=off  OutDataTypeStr=boolean
  Relational Operator : RelationalOperator  OutDataTypeStr=boolean  RndMeth=Simplest
  Relational Operator1 : RelationalOperator  Operator=>  OutDataTypeStr=boolean  RndMeth=Simplest
  Relational Operator3 : RelationalOperator  Operator===  OutDataTypeStr=boolean  RndMeth=Simplest
  DIR_LaneChgRigBySteerValid : Outport
  wires:
  Relational Operator1/1 -> Logical Operator1/3
  Constant1/1 -> Relational Operator1/2
  Logical Operator1/1 -> DIR_LaneChgRigBySteerValid/1  "DIR_LaneChgRigBySteerValid"
  Constant2/1 -> Relational Operator/2
  vxvRefMs/1 -> Relational Operator1/1
  Relational Operator/1 -> Logical Operator1/2
  SteerWheelAngleSign/1 -> Relational Operator3/1
  SteerWheelAngle/1 -> Relational Operator/1
  Relational Operator3/1 -> Logical Operator1/1
  Constant4/1 -> Relational Operator3/2

== system PubIfDecisionLM_MDL/Subsystem2/DIR/DrivingIntentionRecognition1/DIR_LaneChangeProbCalc/DIR_LaneChangeRightProbCalc/If Action Subsystem1/DIR_LaneChgLeProbCalcBySteer/If Action Subsystem1 ==
  SteerWheelAngle : Inport
  SteerWheelAngleSign : Inport  Port=2
  vxvRefMs : Inport  Port=3
  Action Port : ActionPort  ActionPortLabel=else
  1-D Lookup Table : Lookup_n-D  NumberOfTableDimensions=1  BreakpointsForDimension1=single([5,15,25,35]);  Table=single([10,9,6,3]);  InternalRulePriority=Speed  RndMeth=Simplest  InputSameDT=on
  Constant1 : Constant  Value=0  OutDataTypeStr=single
  Constant4 : Constant  OutDataTypeStr=uint8
  Logical Operator1 : Logic  Inputs=3  AllPortsSameDT=off  OutDataTypeStr=boolean
  Relational Operator : RelationalOperator  OutDataTypeStr=boolean  RndMeth=Simplest
  Relational Operator2 : RelationalOperator  Operator=>  OutDataTypeStr=boolean  RndMeth=Simplest
  Relational Operator3 : RelationalOperator  Operator===  OutDataTypeStr=boolean  RndMeth=Simplest
  DIR_LaneChgRigBySteerValid : Outport
  wires:
  Relational Operator2/1 -> Logical Operator1/3
  Constant1/1 -> Relational Operator2/2
  vxvRefMs/1 -> 1-D Lookup Table/1, Relational Operator2/1
  Relational Operator3/1 -> Logical Operator1/1
  Relational Operator/1 -> Logical Operator1/2
  SteerWheelAngle/1 -> Relational Operator/1
  SteerWheelAngleSign/1 -> Relational Operator3/1
  1-D Lookup Table/1 -> Relational Operator/2
  Constant4/1 -> Relational Operator3/2
  Logical Operator1/1 -> DIR_LaneChgRigBySteerValid/1  "DIR_LaneChgRigBySteerValid"

== system PubIfDecisionLM_MDL/Subsystem2/LM_Fusion1/LM_FusRatioCalc/LM_Fusion_EO/LM_FusEVORatioCalc/LM_Fusion_FntPathK/LM_FusEOFntPath1/If Action Subsystem ==
  Action Port : ActionPort  ActionPortLabel=if(u1 == 2)
  Constant : Constant  OutDataTypeStr=single
  Constant1 : Constant  Value=0  OutDataTypeStr=single
  LM_FusEOFntPath1EMLK : Outport
  LM_FusEOFntPath1OTLK : Outport  Port=2
  wires:
  Constant/1 -> LM_FusEOFntPath1EMLK/1  "LM_FusEOFntPath1EMLK"
  Constant1/1 -> LM_FusEOFntPath1OTLK/1  "LM_FusEOFntPath1OTLK"

== system PubIfDecisionLM_MDL/Subsystem2/LM_Fusion1/LM_FusRatioCalc/LM_Fusion_EO/LM_FusEVORatioCalc/LM_Fusion_FntPathK/LM_FusEOFntPath1/If Action Subsystem1 ==
  vxvRefMs : Inport
  LM_EMLFntPath1Quality : Inport  Port=2
  LM_OTLFntPath1Qulity : Inport  Port=3
  Action Port : ActionPort  ActionPortLabel=else
  LM_FusEOFntPath1RatioCalc : Subsystem
  LM_FusEO_EMLFactor : Subsystem
  LM_FusEO_OTLFactor : Subsystem
  LM_FusEOFntPath1EMLK : Outport
  LM_FusEOFntPath1OTLK : Outport  Port=2
  wires:
  LM_FusEO_EMLFactor/1(LM_FusEVOFntPath1EMLFac) -> LM_FusEOFntPath1RatioCalc/2(LM_FusEVOFntPath1EMLFac)
  LM_FusEOFntPath1RatioCalc/2(LM_FusEOFntPath1OTLK) -> LM_FusEOFntPath1OTLK/1
  vxvRefMs/1 -> LM_FusEOFntPath1RatioCalc/1(vxvRefMs), LM_FusEO_EMLFactor/1(vxvRefMs)
  LM_FusEO_OTLFactor/1(LM_FusEVOFntPath1OTLFac) -> LM_FusEOFntPath1RatioCalc/3(LM_FusEVOFntPath1OTLFac)
  LM_FusEOFntPath1RatioCalc/1(LM_FusEOFntPath1EMLK) -> LM_FusEOFntPath1EMLK/1
  LM_OTLFntPath1Qulity/1 -> LM_FusEOFntPath1RatioCalc/5(LM_OTLFntPath1Qulity)
  LM_EMLFntPath1Quality/1 -> LM_FusEOFntPath1RatioCalc/4(LM_EMLFntPath1Quality)

== system PubIfDecisionLM_MDL/Subsystem2/LM_Fusion1/LM_FusRatioCalc/LM_Fusion_EO/LM_FusEVORatioCalc/LM_Fusion_FntPathK/LM_FusEOFntPath2/If Action Subsystem ==
  Action Port : ActionPort  ActionPortLabel=if(u1 == 2)
  Constant : Constant  OutDataTypeStr=single
  Constant1 : Constant  Value=0  OutDataTypeStr=single
  LM_FusEOFntPath2EMLK : Outport
  LM_FusEOFntPath2OTLK : Outport  Port=2
  wires:
  Constant/1 -> LM_FusEOFntPath2EMLK/1  "LM_FusEOFntPath2EMLK"
  Constant1/1 -> LM_FusEOFntPath2OTLK/1  "LM_FusEOFntPath2OTLK"

== system PubIfDecisionLM_MDL/Subsystem2/LM_Fusion1/LM_FusRatioCalc/LM_Fusion_EO/LM_FusEVORatioCalc/LM_Fusion_FntPathK/LM_FusEOFntPath2/If Action Subsystem1 ==
  note: 车速高，第二段EML比例高，OTL比例适当调小
  vxvRefMs : Inport
  LM_EMLFntPath2Quality : Inport  Port=2
  LM_OTLFntPath2Qulity : Inport  Port=3
  Action Port : ActionPort  ActionPortLabel=else
  1-D Lookup Table : Lookup_n-D  NumberOfTableDimensions=1  BreakpointsForDimension1=single([5,10,15,20,35,50,60]);  Table=single([0.10000000149011612,0.15000000596046448,0.20000000298023224,0.4000000059604645,0.5,0.800000011920929,0.949999988079071]);  InternalRulePriority=Speed  RndMeth=Simplest  InputSameDT=on
  Add1 : Sum
  Compare To Zero : simulink/Logic and Bit Operations/Compare To Zero  relop===  OutDataTypeStr=boolean
  Constant : Constant  OutDataTypeStr=single
  Constant1 : Constant  Value=0.55  OutDataTypeStr=single
  Constant2 : Constant  Value=0.5  OutDataTypeStr=single
  Constant3 : Constant  Value=0.000001  OutDataTypeStr=single
  Divide : Product  Inputs=*/
  Divide2 : Product  Inputs=*/
  Product : Product
  Product2 : Product
  Relational Operator : RelationalOperator  OutDataTypeStr=boolean  RndMeth=Simplest
  Subtract : Sum  Inputs=+-
  Switch : Switch  Criteria=u2 ~= 0
  Switch1 : Switch  Criteria=u2 ~= 0
  LM_FusEOFntPath2EMLK : Outport
  LM_FusEOFntPath2OTLK : Outport  Port=2
  wires:
  vxvRefMs/1 -> 1-D Lookup Table/1
  LM_EMLFntPath2Quality/1 -> Product/1
  LM_OTLFntPath2Qulity/1 -> Product2/1, Relational Operator/1
  Divide/1 -> LM_FusEOFntPath2EMLK/1  "LM_FusEOFntPath2EMLK"
  Divide2/1 -> LM_FusEOFntPath2OTLK/1  "LM_FusEOFntPath2OTLK"
  Product/1 -> Add1/1, Divide/1
  Constant/1 -> Subtract/1
  Switch1/1 -> Divide2/2, Divide/2
  Product2/1 -> Divide2/1, Add1/2
  Subtract/1 -> Product2/2
  Relational Operator/1 -> Switch/2
  Constant1/1 -> Relational Operator/2
  1-D Lookup Table/1 -> Switch/1
  Constant2/1 -> Switch/3
  Switch/1 -> Product/2, Subtract/2
  Add1/1 -> Switch1/3, Compare To Zero/1
  Compare To Zero/1 -> Switch1/2
  Constant3/1 -> Switch1/1

== system PubIfDecisionLM_MDL/Subsystem2/LM_Fusion1/LM_FusRatioCalc/LM_Fusion_EO/LM_FusEVORatioCalc/LM_Fusion_FntPathK/LM_FusEOFntPath3/If Action Subsystem ==
  Action Port : ActionPort  ActionPortLabel=if(u1 == 2)
  Constant : Constant  OutDataTypeStr=single
  Constant1 : Constant  Value=0  OutDataTypeStr=single
  LM_FusEOFntPath3EMLK : Outport
  LM_FusEOFntPath3OTLK : Outport  Port=2
  wires:
  Constant/1 -> LM_FusEOFntPath3EMLK/1  "LM_FusEOFntPath3EMLK"
  Constant1/1 -> LM_FusEOFntPath3OTLK/1  "LM_FusEOFntPath3OTLK"

== system PubIfDecisionLM_MDL/Subsystem2/LM_Fusion1/LM_FusRatioCalc/LM_Fusion_EO/LM_FusEVORatioCalc/LM_Fusion_FntPathK/LM_FusEOFntPath3/If Action Subsystem1 ==
  LM_EMLFntPath3Quality : Inport
  LM_OTLFntPath3Qulity : Inport  Port=2
  Action Port : ActionPort  ActionPortLabel=else
  Add1 : Sum
  Compare To Zero : simulink/Logic and Bit Operations/Compare To Zero  relop===  OutDataTypeStr=boolean
  Constant : Constant  Value=0.000001  OutDataTypeStr=single
  Divide : Product  Inputs=*/
  Divide2 : Product  Inputs=*/
  Switch : Switch  Criteria=u2 ~= 0
  LM_FusEOFntPath3EMLK : Outport
  LM_FusEOFntPath3OTLK : Outport  Port=2
  wires:
  LM_EMLFntPath3Quality/1 -> Add1/1, Divide/1
  Switch/1 -> Divide/2, Divide2/2
  LM_OTLFntPath3Qulity/1 -> Divide2/1, Add1/2
  Divide2/1 -> LM_FusEOFntPath3OTLK/1  "LM_FusEOFntPath3OTLK"
  Divide/1 -> LM_FusEOFntPath3EMLK/1  "LM_FusEOFntPath3EMLK"
  Add1/1 -> Switch/3, Compare To Zero/1
  Compare To Zero/1 -> Switch/2
  Constant/1 -> Switch/1

== system PubIfDecisionLM_MDL/Subsystem2/LM_Fusion1/LM_FusRatioCalc/LM_Fusion_EVO/LM_FusEVORatioCalc/LM_Fusion_FntPathK/LM_FusEVOFntPath1/If Action Subsystem1 ==
  LM_VSLFntPath1Quality : Inport
  vxvRefMs : Inport  Port=2
  LM_EMLFntPath1Quality : Inport  Port=3
  LM_OTLFntPath1Qulity : Inport  Port=4
  DIR_LC2LeValid : Inport  Port=5
  DIR_LC2RigValid : Inport  Port=6
  Action Port : ActionPort  ActionPortLabel=else
  LM_FusEVORatioCalc : Subsystem
  LM_FusEVO_EMLFactor : Subsystem
  LM_FusEVO_OTLFactor : Subsystem
  LM_FusEVO_VSLFactor : Subsystem
  LM_FusEVOFntPath1EMLK : Outport
  LM_FusEVOFntPath1VSLK : Outport  Port=2
  LM_FusEVOFntPath1OTLK : Outport  Port=3
  wires:
  vxvRefMs/1 -> LM_FusEVO_EMLFactor/1(vxvRefMs)
  LM_FusEVO_EMLFactor/1(LM_FusEVOFntPath1EMLFac) -> LM_FusEVORatioCalc/1(LM_FusEVOFntPath1EMLFac)
  LM_FusEVO_VSLFactor/1(LM_FusEVOFntPath1VSLFac) -> LM_FusEVORatioCalc/2(LM_FusEVOFntPath1VSLFac)
  LM_FusEVO_OTLFactor/1(LM_FusEVOFntPath1OTLFac) -> LM_FusEVORatioCalc/3(LM_FusEVOFntPath1OTLFac)
  LM_VSLFntPath1Quality/1 -> LM_FusEVORatioCalc/4(LM_VSLFntPath1Quality)
  LM_EMLFntPath1Quality/1 -> LM_FusEVORatioCalc/5(LM_EMLFntPath1Quality)
  LM_OTLFntPath1Qulity/1 -> LM_FusEVORatioCalc/6(LM_OTLFntPath1Qulity)
  LM_FusEVORatioCalc/2(LM_FusEVOFntPath1VSLK) -> LM_FusEVOFntPath1VSLK/1
  LM_FusEVORatioCalc/1(LM_FusEVOFntPath1EMLK) -> LM_FusEVOFntPath1EMLK/1
  LM_FusEVORatioCalc/3(LM_FusEVOFntPath1OTLK) -> LM_FusEVOFntPath1OTLK/1
  DIR_LC2LeValid/1 -> LM_FusEVO_OTLFactor/1(DIR_LC2LeValid), LM_FusEVO_EMLFactor/2(DIR_LC2LeValid)
  DIR_LC2RigValid/1 -> LM_FusEVO_OTLFactor/2(DIR_LC2RigValid), LM_FusEVO_EMLFactor/3(DIR_LC2RigValid)
